simulink model "GDFLIB_FilterFIR_BAM_FLT"  (Simulink 7.3)
settings: Solver=ode45  StartTime=0.0  StopTime=10.0  RelTol=1e-3
undefined symbols (not defined in the file): pfltCoefBuf, u32Order
settings Model: Creator=RE004C  LastModifiedBy=RE004C
settings HardwareCC: ProdIntDivRoundTo=Zero  ProdEndianess=BigEndian  ProdHWDeviceType=Freescale->32-bit PowerPC

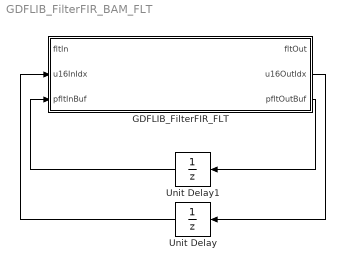
== system GDFLIB_FilterFIR_BAM_FLT ==
  GDFLIB_FilterFIR_FLT : Subsystem  mask(GDFLIB_FilterFIR_FLT){u32Order=u32Order, pfltCoefBuf=pfltCoefBuf}
      mask help: Bit accurate model of FIR filter. All parameters as well as input and output are in single precision floating data format.
      mask init:
      | pos = get_param(gcb, 'Position');width = pos(3) - pos(1); height = pos(4) - pos(2);tX=width/2;tY=height*0.9;
      mask Display:
      | color('black');
      | port_label('input',1,'fltIn');
      | port_label('input',2,'u16InIdx');
      | port_label('input',3,'pfltInBuf');
      | port_label('output',1,'fltOut');
      | port_label('output',2,'u16OutIdx');
      | port_label('output',3,'pfltOutBuf');
      | color('black');
      | disp('GDFLIB_FilterFIR_FLT');
      | color('blue');
      | text(tX,tY, 'BAM', 'horizontalAlignment', 'center');
  Unit Delay : UnitDelay  SampleTime=-1
  Unit Delay1 : UnitDelay  SampleTime=-1
  wires:
  GDFLIB_FilterFIR_FLT/2(u16OutIdx) -> Unit Delay/1
  Unit Delay/1 -> GDFLIB_FilterFIR_FLT/2(u16InIdx)
  GDFLIB_FilterFIR_FLT/3(pfltOutBuf) -> Unit Delay1/1
  Unit Delay1/1 -> GDFLIB_FilterFIR_FLT/3(pfltInBuf)

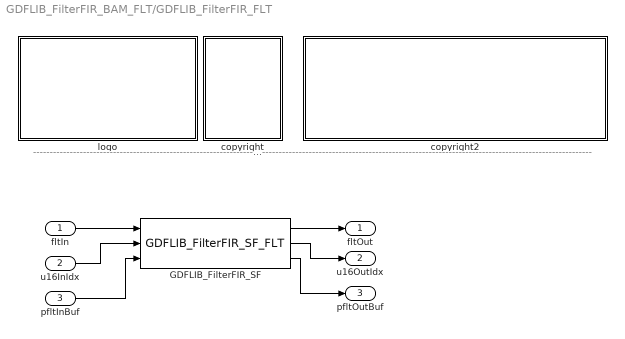
== system GDFLIB_FilterFIR_BAM_FLT/GDFLIB_FilterFIR_FLT ==
  note: ---------------------------------------------------------------------------------------------------------------------------------------------------------------------------------------------------
  fltIn : Inport  OutDataType=fixdt(1, 16)  OutScaling=2^0
  u16InIdx : Inport  Port=2  OutDataType=fixdt(1, 16)  OutScaling=2^0
  pfltInBuf : Inport  Port=3  OutDataType=fixdt(1, 16)  OutScaling=2^0
  GDFLIB_FilterFIR_SF : S-Function  FunctionName=GDFLIB_FilterFIR_SF_FLT  Parameters=u32Order,pfltCoefBuf  EnableBusSupport=off
  copyright : Subsystem
      mask Display: text(10,90,'FILE:');text(10,75,'DESRIPTION:')text(10,60,'COPYRIGHT:')text(10,45,'VERSION:')text(10,30,'DATE:')
  copyright2 : Subsystem
      mask Display: text(10,90,'GDFLIB_FilterFIR_BAM_FLT.mdl');text(10,75,'FIR filter.');text(10,60,'Freescale')text(10,45,'0.1');text(10,30,'20-Sep-2011');
  logo : Subsystem
      mask Display: image(imread('logo.jpg'))
  fltOut : Outport  OutDataType=fixdt(1, 16)  OutScaling=2^0
  u16OutIdx : Outport  Port=2  OutDataType=fixdt(1, 16)  OutScaling=2^0
  pfltOutBuf : Outport  Port=3  OutDataType=fixdt(1, 16)  OutScaling=2^0
  wires:
  fltIn/1 -> GDFLIB_FilterFIR_SF/1
  GDFLIB_FilterFIR_SF/1 -> fltOut/1
  u16InIdx/1 -> GDFLIB_FilterFIR_SF/2
  pfltInBuf/1 -> GDFLIB_FilterFIR_SF/3
  GDFLIB_FilterFIR_SF/2 -> u16OutIdx/1
  GDFLIB_FilterFIR_SF/3 -> pfltOutBuf/1

== system GDFLIB_FilterFIR_BAM_FLT/GDFLIB_FilterFIR_FLT/copyright ==

== system GDFLIB_FilterFIR_BAM_FLT/GDFLIB_FilterFIR_FLT/copyright2 ==

== system GDFLIB_FilterFIR_BAM_FLT/GDFLIB_FilterFIR_FLT/logo ==
